simulink model "SF054A_PwrpkCmpbltyChk"  (R2013b)
settings: Solver=FixedStepDiscrete  SolverMode=SingleTasking  StartTime=0.0  StopTime=1  FixedStep=0.1  RelTol=1e-3
values from neighbouring files (symbols this model uses):
  CNVTOCNT_CNTPERMILLISEC_U32 = DataDict.Constant    [SF054A_PwrpkCmpbltyChk_DataDict.m]
  CORRLNFLTBIT2_CNT_U08 = DataDict.Constant    [SF054A_PwrpkCmpbltyChk_DataDict.m]
  CORRLNGEARIDFLTBIT3_CNT_U08 = DataDict.Constant    [SF054A_PwrpkCmpbltyChk_DataDict.m]
  GEARID1INVLBIT0_CNT_U08 = DataDict.Constant    [SF054A_PwrpkCmpbltyChk_DataDict.m]
  GEARID2INVLBIT1_CNT_U08 = DataDict.Constant    [SF054A_PwrpkCmpbltyChk_DataDict.m]
  NODEBSTEP_CNT_U16 = DataDict.Constant    [SF054A_PwrpkCmpbltyChk_DataDict.m]
  NOFAULT_CNT_U08 = DataDict.Constant    [SF054A_PwrpkCmpbltyChk_DataDict.m]
  PwrpkCmpbltyChkGearId = DataDict.Calibration    [SF054A_PwrpkCmpbltyChk_DataDict.m]
  TMRTHD_MILLISEC_U32 = DataDict.Constant    [SF054A_PwrpkCmpbltyChk_DataDict.m]
undefined symbols (not defined in the file or in its folder): NtcNr1, NtcSts1, SigQlfr1
libraries: simulink x10
(part 3 of 3)

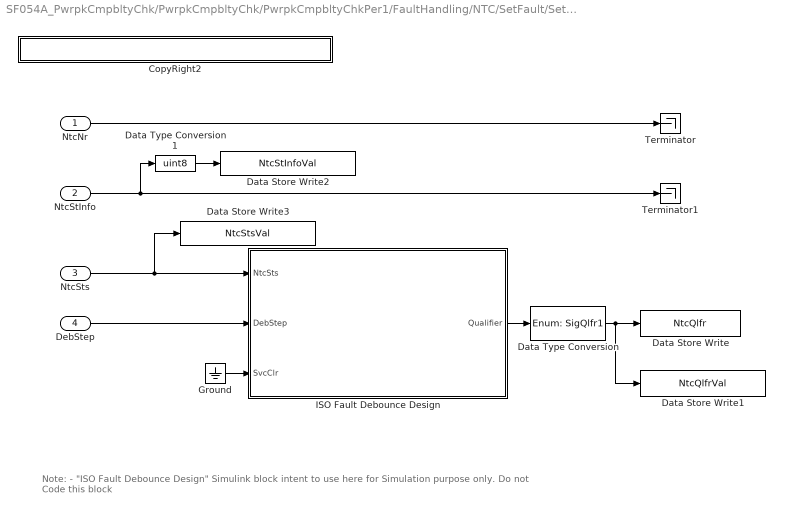
== system SF054A_PwrpkCmpbltyChk/PwrpkCmpbltyChk/PwrpkCmpbltyChkPer1/FaultHandling/NTC/SetFault/SetNtcSts ==
  note: Note:
      |
      | - "ISO Fault Debounce Design" Simulink block intent to use here for Simulation purpose only. Do not Code this block
  NtcNr : Inport
  NtcStInfo : Inport  Port=2
  NtcSts : Inport  Port=3
  DebStep : Inport  Port=4
  CopyRight2 : Subsystem  Description=|  mask(Copyright Information){none=on}
      | Copyright info block.                                               
      |                                                                     
      | Place copyright information at the top of every subsystem in design.
      mask prompts: none "No parameters"
      mask help: Place copyright information at the top of every subsystem in design.
      mask Display:
      | NxtrConf = 'Nexteer Confidential';
      | 
      | sys = bdroot; %handle for the current model ("system")
      | first = get_param(sys,'Created');
      | if(isempty(first))
      |     first = datestr(now,'yyyy');
      | else
      |     first = first(end-3:end);  %year is last four digits
      | end
      | 
      | last = get_param(sys,'LastModifiedDate');
      | if isempty(last)
      |     last = datestr(now,'yyyy');
      | else
      |     last = last(end-3:end);
      | end
      | 
      | if strcmp(first,last)
      |     fprintf('%s -- Copyright %s Nexteer',NxtrConf,first)
      | else
      |     fprintf('%s -- %s%s- %s Nexteer',NxtrConf,char(169),first,last)
      | end
  Data Store Write : DataStoreWrite  DataStoreName=NtcQlfr
  Data Store Write1 : DataStoreWrite  DataStoreName=NtcQlfrVal
  Data Store Write2 : DataStoreWrite  DataStoreName=NtcStInfoVal
  Data Store Write3 : DataStoreWrite  DataStoreName=NtcStsVal
  Data Type Conversion : DataTypeConversion  OutDataTypeStr=Enum: SigQlfr1
  Data Type Conversion1 : DataTypeConversion  OutDataTypeStr=uint8
  Ground : Ground
  ISO Fault Debounce Design : Stateflow chart  TreatAsAtomicUnit=on
      settings: AttributesFormatString=|
      | Simulation Purpose Only.
      | Do Not Code this block
      | Diagnostic Manager Owns this requirement
  Terminator : Terminator
  Terminator1 : Terminator
  wires:
  NtcNr/1 -> Terminator/1
  DebStep/1 -> ISO Fault Debounce Design/2(DebStep)
  ISO Fault Debounce Design/1(Qualifier) -> Data Type Conversion/1
  Ground/1 -> ISO Fault Debounce Design/3(SvcClr)
  Data Type Conversion/1 -> Data Store Write1/1, Data Store Write/1
  NtcSts/1 -> Data Store Write3/1, ISO Fault Debounce Design/1(NtcSts)
  NtcStInfo/1 -> Data Type Conversion1/1, Terminator1/1
  Data Type Conversion1/1 -> Data Store Write2/1

== system SF054A_PwrpkCmpbltyChk/PwrpkCmpbltyChk/PwrpkCmpbltyChkPer1/FaultHandling/NTCCheck/GetNtcQlfrSts/CopyRight2 ==

== system SF054A_PwrpkCmpbltyChk/PwrpkCmpbltyChk/PwrpkCmpbltyChkPer1/FaultDetection/CorrlnChk/CorrlnFltChk/GearIdCorrlnChk/CopyRight2 ==

== system SF054A_PwrpkCmpbltyChk/PwrpkCmpbltyChk/PwrpkCmpbltyChkPer1/FaultDetection/CorrlnChk/CorrlnFltChk/GearIdCorrlnChk/Default ==
  Action Port : ActionPort  ActionType=else
  Constant1 : Constant  Value=true  OutDataTypeStr=boolean
      settings: AttributesFormatString=%<OutDataTypeStr>
  Constant7 : Constant  Value=CORRLNGEARIDFLTBIT3_CNT_U08
  CopyRight2 : Subsystem  Description=|  mask(Copyright Information){none=on}
      | Copyright info block.                                               
      |                                                                     
      | Place copyright information at the top of every subsystem in design.
      mask prompts: none "No parameters"
      mask help: Place copyright information at the top of every subsystem in design.
      mask Display:
      | NxtrConf = 'Nexteer Confidential';
      | 
      | sys = bdroot; %handle for the current model ("system")
      | first = get_param(sys,'Created');
      | if(isempty(first))
      |     first = datestr(now,'yyyy');
      | else
      |     first = first(end-3:end);  %year is last four digits
      | end
      | 
      | last = get_param(sys,'LastModifiedDate');
      | if isempty(last)
      |     last = datestr(now,'yyyy');
      | else
      |     last = last(end-3:end);
      | end
      | 
      | if strcmp(first,last)
      |     fprintf('%s -- Copyright %s Nexteer',NxtrConf,first)
      | else
      |     fprintf('%s -- %s%s- %s Nexteer',NxtrConf,char(169),first,last)
      | end
  GearIdCorrlnFltCnt : Outport
  GearIdCorrlnFltStat : Outport  Port=2
  wires:
  Constant1/1 -> GearIdCorrlnFltStat/1
  Constant7/1 -> GearIdCorrlnFltCnt/1

== system SF054A_PwrpkCmpbltyChk/PwrpkCmpbltyChk/PwrpkCmpbltyChkPer1/FaultDetection/CorrlnChk/CorrlnFltChk/GearIdCorrlnChk/GearIdCorlnChk ==
  Action Port : ActionPort  ActionType=then
  Constant2 : Constant  Value=NOFAULT_CNT_U08
  Constant4 : Constant  Value=false  OutDataTypeStr=boolean
      settings: AttributesFormatString=%<OutDataTypeStr>
  CopyRight2 : Subsystem  Description=|  mask(Copyright Information){none=on}
      | Copyright info block.                                               
      |                                                                     
      | Place copyright information at the top of every subsystem in design.
      mask prompts: none "No parameters"
      mask help: Place copyright information at the top of every subsystem in design.
      mask Display:
      | NxtrConf = 'Nexteer Confidential';
      | 
      | sys = bdroot; %handle for the current model ("system")
      | first = get_param(sys,'Created');
      | if(isempty(first))
      |     first = datestr(now,'yyyy');
      | else
      |     first = first(end-3:end);  %year is last four digits
      | end
      | 
      | last = get_param(sys,'LastModifiedDate');
      | if isempty(last)
      |     last = datestr(now,'yyyy');
      | else
      |     last = last(end-3:end);
      | end
      | 
      | if strcmp(first,last)
      |     fprintf('%s -- Copyright %s Nexteer',NxtrConf,first)
      | else
      |     fprintf('%s -- %s%s- %s Nexteer',NxtrConf,char(169),first,last)
      | end
  GearIdCorrlnFltStat : Outport
  GearIdCorrlnFltCnt : Outport  Port=2
  wires:
  Constant4/1 -> GearIdCorrlnFltStat/1
  Constant2/1 -> GearIdCorrlnFltCnt/1

== system SF054A_PwrpkCmpbltyChk/PwrpkCmpbltyChk/PwrpkCmpbltyChkPer1/FaultDetection/CorrlnChk/CorrlnFltChk/SigCorrlnChk/CopyRight2 ==

== system SF054A_PwrpkCmpbltyChk/PwrpkCmpbltyChk/PwrpkCmpbltyChkPer1/FaultDetection/CorrlnChk/CorrlnFltChk/SigCorrlnChk/CorrelationCheck ==
  Action Port : ActionPort  ActionType=then
  Constant1 : Constant  Value=NOFAULT_CNT_U08
  Constant4 : Constant  Value=false  OutDataTypeStr=boolean
      settings: AttributesFormatString=%<OutDataTypeStr>
  CopyRight2 : Subsystem  Description=|  mask(Copyright Information){none=on}
      | Copyright info block.                                               
      |                                                                     
      | Place copyright information at the top of every subsystem in design.
      mask prompts: none "No parameters"
      mask help: Place copyright information at the top of every subsystem in design.
      mask Display:
      | NxtrConf = 'Nexteer Confidential';
      | 
      | sys = bdroot; %handle for the current model ("system")
      | first = get_param(sys,'Created');
      | if(isempty(first))
      |     first = datestr(now,'yyyy');
      | else
      |     first = first(end-3:end);  %year is last four digits
      | end
      | 
      | last = get_param(sys,'LastModifiedDate');
      | if isempty(last)
      |     last = datestr(now,'yyyy');
      | else
      |     last = last(end-3:end);
      | end
      | 
      | if strcmp(first,last)
      |     fprintf('%s -- Copyright %s Nexteer',NxtrConf,first)
      | else
      |     fprintf('%s -- %s%s- %s Nexteer',NxtrConf,char(169),first,last)
      | end
  CorrlnFltStat : Outport
  CorrlnFltCnt : Outport  Port=2
  wires:
  Constant4/1 -> CorrlnFltStat/1
  Constant1/1 -> CorrlnFltCnt/1

== system SF054A_PwrpkCmpbltyChk/PwrpkCmpbltyChk/PwrpkCmpbltyChkPer1/FaultDetection/CorrlnChk/CorrlnFltChk/SigCorrlnChk/Default ==
  Action Port : ActionPort  ActionType=else
  Constant2 : Constant  Value=true  OutDataTypeStr=boolean
      settings: AttributesFormatString=%<OutDataTypeStr>
  Constant5 : Constant  Value=CORRLNFLTBIT2_CNT_U08
  CopyRight2 : Subsystem  Description=|  mask(Copyright Information){none=on}
      | Copyright info block.                                               
      |                                                                     
      | Place copyright information at the top of every subsystem in design.
      mask prompts: none "No parameters"
      mask help: Place copyright information at the top of every subsystem in design.
      mask Display:
      | NxtrConf = 'Nexteer Confidential';
      | 
      | sys = bdroot; %handle for the current model ("system")
      | first = get_param(sys,'Created');
      | if(isempty(first))
      |     first = datestr(now,'yyyy');
      | else
      |     first = first(end-3:end);  %year is last four digits
      | end
      | 
      | last = get_param(sys,'LastModifiedDate');
      | if isempty(last)
      |     last = datestr(now,'yyyy');
      | else
      |     last = last(end-3:end);
      | end
      | 
      | if strcmp(first,last)
      |     fprintf('%s -- Copyright %s Nexteer',NxtrConf,first)
      | else
      |     fprintf('%s -- %s%s- %s Nexteer',NxtrConf,char(169),first,last)
      | end
  CorrlnFltCnt : Outport
  CorrlnFltStat : Outport  Port=2
  wires:
  Constant2/1 -> CorrlnFltStat/1
  Constant5/1 -> CorrlnFltCnt/1

== system SF054A_PwrpkCmpbltyChk/PwrpkCmpbltyChk/PwrpkCmpbltyChkPer1/FaultDetection/GearSigChk/GearSigVldChk/GearIdn1/CopyRight2 ==

== system SF054A_PwrpkCmpbltyChk/PwrpkCmpbltyChk/PwrpkCmpbltyChkPer1/FaultDetection/GearSigChk/GearSigVldChk/GearIdn1/Default ==
  Action Port : ActionPort  ActionType=else
  Constant1 : Constant  Value=true  OutDataTypeStr=boolean
      settings: AttributesFormatString=%<OutDataTypeStr>
  Constant2 : Constant  Value=false  OutDataTypeStr=boolean
      settings: AttributesFormatString=%<OutDataTypeStr>
  Constant6 : Constant  Value=GEARID1INVLBIT0_CNT_U08  OutDataTypeStr=uint8
      settings: AttributesFormatString=%<OutDataTypeStr>
  CopyRight2 : Subsystem  Description=|  mask(Copyright Information){none=on}
      | Copyright info block.                                               
      |                                                                     
      | Place copyright information at the top of every subsystem in design.
      mask prompts: none "No parameters"
      mask help: Place copyright information at the top of every subsystem in design.
      mask Display:
      | NxtrConf = 'Nexteer Confidential';
      | 
      | sys = bdroot; %handle for the current model ("system")
      | first = get_param(sys,'Created');
      | if(isempty(first))
      |     first = datestr(now,'yyyy');
      | else
      |     first = first(end-3:end);  %year is last four digits
      | end
      | 
      | last = get_param(sys,'LastModifiedDate');
      | if isempty(last)
      |     last = datestr(now,'yyyy');
      | else
      |     last = last(end-3:end);
      | end
      | 
      | if strcmp(first,last)
      |     fprintf('%s -- Copyright %s Nexteer',NxtrConf,first)
      | else
      |     fprintf('%s -- %s%s- %s Nexteer',NxtrConf,char(169),first,last)
      | end
  GearIdn1FltCnt : Outport
  GearIdn1FltStat : Outport  Port=2
  GearIdn1VldStat : Outport  Port=3
  wires:
  Constant2/1 -> GearIdn1VldStat/1
  Constant1/1 -> GearIdn1FltStat/1
  Constant6/1 -> GearIdn1FltCnt/1

== system SF054A_PwrpkCmpbltyChk/PwrpkCmpbltyChk/PwrpkCmpbltyChkPer1/FaultDetection/GearSigChk/GearSigVldChk/GearIdn1/GearId1Vld ==
  Action Port : ActionPort  ActionType=then
  Constant1 : Constant  Value=true  OutDataTypeStr=boolean
      settings: AttributesFormatString=%<OutDataTypeStr>
  Constant2 : Constant  Value=false  OutDataTypeStr=boolean
      settings: AttributesFormatString=%<OutDataTypeStr>
  Constant3 : Constant  Value=NOFAULT_CNT_U08  OutDataTypeStr=uint8
      settings: AttributesFormatString=%<OutDataTypeStr>
  CopyRight2 : Subsystem  Description=|  mask(Copyright Information){none=on}
      | Copyright info block.                                               
      |                                                                     
      | Place copyright information at the top of every subsystem in design.
      mask prompts: none "No parameters"
      mask help: Place copyright information at the top of every subsystem in design.
      mask Display:
      | NxtrConf = 'Nexteer Confidential';
      | 
      | sys = bdroot; %handle for the current model ("system")
      | first = get_param(sys,'Created');
      | if(isempty(first))
      |     first = datestr(now,'yyyy');
      | else
      |     first = first(end-3:end);  %year is last four digits
      | end
      | 
      | last = get_param(sys,'LastModifiedDate');
      | if isempty(last)
      |     last = datestr(now,'yyyy');
      | else
      |     last = last(end-3:end);
      | end
      | 
      | if strcmp(first,last)
      |     fprintf('%s -- Copyright %s Nexteer',NxtrConf,first)
      | else
      |     fprintf('%s -- %s%s- %s Nexteer',NxtrConf,char(169),first,last)
      | end
  GearIdn1VldStat : Outport
  GearIdn1FltStat : Outport  Port=2
  GearIdn1FltCnt : Outport  Port=3
  wires:
  Constant1/1 -> GearIdn1VldStat/1
  Constant2/1 -> GearIdn1FltStat/1
  Constant3/1 -> GearIdn1FltCnt/1

== system SF054A_PwrpkCmpbltyChk/PwrpkCmpbltyChk/PwrpkCmpbltyChkPer1/FaultDetection/GearSigChk/GearSigVldChk/GearIdn2/CopyRight2 ==

== system SF054A_PwrpkCmpbltyChk/PwrpkCmpbltyChk/PwrpkCmpbltyChkPer1/FaultDetection/GearSigChk/GearSigVldChk/GearIdn2/Default ==
  Action Port : ActionPort  ActionType=else
  Constant1 : Constant  Value=true  OutDataTypeStr=boolean
      settings: AttributesFormatString=%<OutDataTypeStr>
  Constant2 : Constant  Value=false  OutDataTypeStr=boolean
      settings: AttributesFormatString=%<OutDataTypeStr>
  Constant6 : Constant  Value=GEARID2INVLBIT1_CNT_U08  OutDataTypeStr=uint8
      settings: AttributesFormatString=%<OutDataTypeStr>
  CopyRight2 : Subsystem  Description=|  mask(Copyright Information){none=on}
      | Copyright info block.                                               
      |                                                                     
      | Place copyright information at the top of every subsystem in design.
      mask prompts: none "No parameters"
      mask help: Place copyright information at the top of every subsystem in design.
      mask Display:
      | NxtrConf = 'Nexteer Confidential';
      | 
      | sys = bdroot; %handle for the current model ("system")
      | first = get_param(sys,'Created');
      | if(isempty(first))
      |     first = datestr(now,'yyyy');
      | else
      |     first = first(end-3:end);  %year is last four digits
      | end
      | 
      | last = get_param(sys,'LastModifiedDate');
      | if isempty(last)
      |     last = datestr(now,'yyyy');
      | else
      |     last = last(end-3:end);
      | end
      | 
      | if strcmp(first,last)
      |     fprintf('%s -- Copyright %s Nexteer',NxtrConf,first)
      | else
      |     fprintf('%s -- %s%s- %s Nexteer',NxtrConf,char(169),first,last)
      | end
  GearIdn2FltCnt : Outport
  GearIdn2FltStat : Outport  Port=2
  GearIdn2VldStat : Outport  Port=3
  wires:
  Constant6/1 -> GearIdn2FltCnt/1
  Constant1/1 -> GearIdn2FltStat/1
  Constant2/1 -> GearIdn2VldStat/1

== system SF054A_PwrpkCmpbltyChk/PwrpkCmpbltyChk/PwrpkCmpbltyChkPer1/FaultDetection/GearSigChk/GearSigVldChk/GearIdn2/GearId1Vld ==
  Action Port : ActionPort  ActionType=then
  Constant1 : Constant  Value=true  OutDataTypeStr=boolean
      settings: AttributesFormatString=%<OutDataTypeStr>
  Constant2 : Constant  Value=false  OutDataTypeStr=boolean
      settings: AttributesFormatString=%<OutDataTypeStr>
  Constant3 : Constant  Value=NOFAULT_CNT_U08  OutDataTypeStr=uint8
      settings: AttributesFormatString=%<OutDataTypeStr>
  CopyRight2 : Subsystem  Description=|  mask(Copyright Information){none=on}
      | Copyright info block.                                               
      |                                                                     
      | Place copyright information at the top of every subsystem in design.
      mask prompts: none "No parameters"
      mask help: Place copyright information at the top of every subsystem in design.
      mask Display:
      | NxtrConf = 'Nexteer Confidential';
      | 
      | sys = bdroot; %handle for the current model ("system")
      | first = get_param(sys,'Created');
      | if(isempty(first))
      |     first = datestr(now,'yyyy');
      | else
      |     first = first(end-3:end);  %year is last four digits
      | end
      | 
      | last = get_param(sys,'LastModifiedDate');
      | if isempty(last)
      |     last = datestr(now,'yyyy');
      | else
      |     last = last(end-3:end);
      | end
      | 
      | if strcmp(first,last)
      |     fprintf('%s -- Copyright %s Nexteer',NxtrConf,first)
      | else
      |     fprintf('%s -- %s%s- %s Nexteer',NxtrConf,char(169),first,last)
      | end
  GearIdn2VldStat : Outport
  GearIdn2FltStat : Outport  Port=2
  GearIdn2FltCnt : Outport  Port=3
  wires:
  Constant3/1 -> GearIdn2FltCnt/1
  Constant2/1 -> GearIdn2FltStat/1
  Constant1/1 -> GearIdn2VldStat/1

== system SF054A_PwrpkCmpbltyChk/PwrpkCmpbltyChk/PwrpkCmpbltyChkPer1/FaultDetection/GearSigChk/TmrElpdDetn/GetTiSpan100MicroSec32bit/CopyRight2 ==

== system SF054A_PwrpkCmpbltyChk/PwrpkCmpbltyChk/PwrpkCmpbltyChkPer1/FaultDetection/GearSigChk/TmrElpdDetn/GetTiSpan100MicroSec32bit/No wrapping ==
  new : Inport
  ref : Inport  Port=2
  Action Port : ActionPort  ActionType=then
  CopyRight2 : Subsystem  Description=|  mask(Copyright Information){none=on}
      | Copyright info block.                                               
      |                                                                     
      | Place copyright information at the top of every subsystem in design.
      mask prompts: none "No parameters"
      mask help: Place copyright information at the top of every subsystem in design.
      mask Display:
      | NxtrConf = 'Nexteer Confidential';
      | 
      | sys = bdroot; %handle for the current model ("system")
      | first = get_param(sys,'Created');
      | if(isempty(first))
      |     first = datestr(now,'yyyy');
      | else
      |     first = first(end-3:end);  %year is last four digits
      | end
      | 
      | last = get_param(sys,'LastModifiedDate');
      | if isempty(last)
      |     last = datestr(now,'yyyy');
      | else
      |     last = last(end-3:end);
      | end
      | 
      | if strcmp(first,last)
      |     fprintf('%s -- Copyright %s Nexteer',NxtrConf,first)
      | else
      |     fprintf('%s -- %s%s- %s Nexteer',NxtrConf,char(169),first,last)
      | end
  Subtract1 : Sum  Inputs=+-
  Out1 : Outport
  wires:
  ref/1 -> Subtract1/2
  new/1 -> Subtract1/1
  Subtract1/1 -> Out1/1

== system SF054A_PwrpkCmpbltyChk/PwrpkCmpbltyChk/PwrpkCmpbltyChkPer1/FaultDetection/GearSigChk/TmrElpdDetn/GetTiSpan100MicroSec32bit/Wrapping ==
  new : Inport
  ref : Inport  Port=2
  Action Port : ActionPort  ActionType=else
  CopyRight2 : Subsystem  Description=|  mask(Copyright Information){none=on}
      | Copyright info block.                                               
      |                                                                     
      | Place copyright information at the top of every subsystem in design.
      mask prompts: none "No parameters"
      mask help: Place copyright information at the top of every subsystem in design.
      mask Display:
      | NxtrConf = 'Nexteer Confidential';
      | 
      | sys = bdroot; %handle for the current model ("system")
      | first = get_param(sys,'Created');
      | if(isempty(first))
      |     first = datestr(now,'yyyy');
      | else
      |     first = first(end-3:end);  %year is last four digits
      | end
      | 
      | last = get_param(sys,'LastModifiedDate');
      | if isempty(last)
      |     last = datestr(now,'yyyy');
      | else
      |     last = last(end-3:end);
      | end
      | 
      | if strcmp(first,last)
      |     fprintf('%s -- Copyright %s Nexteer',NxtrConf,first)
      | else
      |     fprintf('%s -- %s%s- %s Nexteer',NxtrConf,char(169),first,last)
      | end
  Max Counts : Constant  Value=2^32-1  OutDataTypeStr=uint32
  Subtract1 : Sum  Inputs=+-+
  Out1 : Outport
  wires:
  new/1 -> Subtract1/3
  ref/1 -> Subtract1/2
  Max Counts/1 -> Subtract1/1
  Subtract1/1 -> Out1/1

== system SF054A_PwrpkCmpbltyChk/PwrpkCmpbltyChk/PwrpkCmpbltyChkPer1/FaultHandling/NTC/NoFault/SetNtcSts/CopyRight2 ==

== system SF054A_PwrpkCmpbltyChk/PwrpkCmpbltyChk/PwrpkCmpbltyChkPer1/FaultHandling/NTC/SetFault/SetNtcSts/CopyRight2 ==

== system SF054A_PwrpkCmpbltyChk/PwrpkCmpbltyChk/PwrpkCmpbltyChkPer1/FaultDetection/CorrlnChk/CorrlnFltChk/GearIdCorrlnChk/Default/CopyRight2 ==

== system SF054A_PwrpkCmpbltyChk/PwrpkCmpbltyChk/PwrpkCmpbltyChkPer1/FaultDetection/CorrlnChk/CorrlnFltChk/GearIdCorrlnChk/GearIdCorlnChk/CopyRight2 ==

== system SF054A_PwrpkCmpbltyChk/PwrpkCmpbltyChk/PwrpkCmpbltyChkPer1/FaultDetection/CorrlnChk/CorrlnFltChk/SigCorrlnChk/CorrelationCheck/CopyRight2 ==

== system SF054A_PwrpkCmpbltyChk/PwrpkCmpbltyChk/PwrpkCmpbltyChkPer1/FaultDetection/CorrlnChk/CorrlnFltChk/SigCorrlnChk/Default/CopyRight2 ==

== system SF054A_PwrpkCmpbltyChk/PwrpkCmpbltyChk/PwrpkCmpbltyChkPer1/FaultDetection/GearSigChk/GearSigVldChk/GearIdn1/Default/CopyRight2 ==

== system SF054A_PwrpkCmpbltyChk/PwrpkCmpbltyChk/PwrpkCmpbltyChkPer1/FaultDetection/GearSigChk/GearSigVldChk/GearIdn1/GearId1Vld/CopyRight2 ==

== system SF054A_PwrpkCmpbltyChk/PwrpkCmpbltyChk/PwrpkCmpbltyChkPer1/FaultDetection/GearSigChk/GearSigVldChk/GearIdn2/Default/CopyRight2 ==

== system SF054A_PwrpkCmpbltyChk/PwrpkCmpbltyChk/PwrpkCmpbltyChkPer1/FaultDetection/GearSigChk/GearSigVldChk/GearIdn2/GearId1Vld/CopyRight2 ==

== system SF054A_PwrpkCmpbltyChk/PwrpkCmpbltyChk/PwrpkCmpbltyChkPer1/FaultDetection/GearSigChk/TmrElpdDetn/GetTiSpan100MicroSec32bit/No wrapping/CopyRight2 ==

== system SF054A_PwrpkCmpbltyChk/PwrpkCmpbltyChk/PwrpkCmpbltyChkPer1/FaultDetection/GearSigChk/TmrElpdDetn/GetTiSpan100MicroSec32bit/Wrapping/CopyRight2 ==

== stateflow chart SF054A_PwrpkCmpbltyChk/PwrpkCmpbltyChk/PwrpkCmpbltyChkPer1/FaultHandling/NTC/NoFault/SetNtcSts/ISO Fault Debounce Design ==
  note: NTCSTS_PASSD           (0)
      | NTCSTS_FAILD             (1)
      | NTCSTS_PREPASSD   (2)
      | NTCSTS_PREFAILD     (3)
      |
      | SIGQLFR_NORES        (0)
      | SIGQLFR_PASSD         (1)
      | SIGQLFR_FAILD           (2)
  note: Pass Loop
  note: Fail Loop
  note: 
  (default) -> (junction 89)
  (junction 89) -> (junction 95) [order 1] : [NtcSts ==3]
  (junction 89) -> (junction 93) [order 2] : [NtcSts ==2]
  (junction 89) -> (junction 141) [order 3] : [NtcSts ==1]
      | { ErrAcc = 32767;
      | Qualifier =2;
      |  }
  (junction 89) -> (junction 141) [order 4] : [NtcSts ==0]
      | { ErrAcc = -32768;
      | Qualifier=1;
      | }
  (junction 95) -> (junction 103) [order 2]
  (junction 95) -> (junction 111) [order 1] : [ErrAcc <=0]
      | {ErrAcc = DebStep;}
  (junction 93) -> (junction 123) [order 2] : {
      | ErrAcc = ErrAcc - DebStep;
      | }
  (junction 93) -> (junction 123) [order 1] : [(ErrAcc - DebStep) <= -32768]
      | { ErrAcc = -32768;
      | Qualifier=1;
      | }
  (junction 103) -> (junction 111) [order 1] : [(ErrAcc + DebStep) <32767]
      | {ErrAcc = ErrAcc + DebStep;}
  (junction 103) -> (junction 111) [order 2] : {ErrAcc = 32767;
      | Qualifier =2;}
  (junction 123) -> (junction 141)
  (junction 111) -> (junction 141)
  (junction 141) -> (junction 159) [order 2] : {ErrAcc = 0;
      | Qualifier =0;
      | }
  (junction 141) -> (junction 159) [order 1] : [SvcClr ==0]
  data: NtcSts input Enum: NtcSts1; Qualifier output uint8; DebStep input uint16; ErrAcc local single; SvcClr input

== stateflow chart SF054A_PwrpkCmpbltyChk/PwrpkCmpbltyChk/PwrpkCmpbltyChkPer1/FaultHandling/NTC/SetFault/SetNtcSts/ISO Fault Debounce Design ==
  note: NTCSTS_PASSD           (0)
      | NTCSTS_FAILD             (1)
      | NTCSTS_PREPASSD   (2)
      | NTCSTS_PREFAILD     (3)
      |
      | SIGQLFR_NORES        (0)
      | SIGQLFR_PASSD         (1)
      | SIGQLFR_FAILD           (2)
  note: Pass Loop
  note: Fail Loop
  note: 
  (default) -> (junction 89)
  (junction 89) -> (junction 95) [order 1] : [NtcSts ==3]
  (junction 89) -> (junction 93) [order 2] : [NtcSts ==2]
  (junction 89) -> (junction 141) [order 3] : [NtcSts ==1]
      | { ErrAcc = 32767;
      | Qualifier =2;
      |  }
  (junction 89) -> (junction 141) [order 4] : [NtcSts ==0]
      | { ErrAcc = -32768;
      | Qualifier=1;
      | }
  (junction 95) -> (junction 103) [order 2]
  (junction 95) -> (junction 111) [order 1] : [ErrAcc <=0]
      | {ErrAcc = DebStep;}
  (junction 93) -> (junction 123) [order 2] : {
      | ErrAcc = ErrAcc - DebStep;
      | }
  (junction 93) -> (junction 123) [order 1] : [(ErrAcc - DebStep) <= -32768]
      | { ErrAcc = -32768;
      | Qualifier=1;
      | }
  (junction 103) -> (junction 111) [order 1] : [(ErrAcc + DebStep) <32767]
      | {ErrAcc = ErrAcc + DebStep;}
  (junction 103) -> (junction 111) [order 2] : {ErrAcc = 32767;
      | Qualifier =2;}
  (junction 123) -> (junction 141)
  (junction 111) -> (junction 141)
  (junction 141) -> (junction 159) [order 2] : {ErrAcc = 0;
      | Qualifier =0;
      | }
  (junction 141) -> (junction 159) [order 1] : [SvcClr ==0]
  data: NtcSts input Enum: NtcSts1; Qualifier output uint8; DebStep input uint16; ErrAcc local single; SvcClr input
